simulink model "controllo_Completo_v14"  (R2025a)
settings: Solver=VariableStepAuto  StartTime=0.0  StopTime=Durata_Simulazione  MaxStep=Passo_integrazione_massimo  RelTol=1e-3
values from neighbouring files (symbols this model uses):
  C_bat_eq_rx = 1.0    (= 1)    [p_schema_completo_generale_v2.m]
  C_bat_eq_tx = 3.5    [p_schema_completo_generale_v2.m]
  C_bus_dc_dc = 1.5e-3    (= 0.0015)    [p_schema_completo_generale_v2.m]
  C_ris = 1/(w_dc_ac_nom^2*L_coil)    (= 6.49245057301e-08)    [p_schema_completo_generale_v2.m]
  dead_time_dc_dc = 0.3e-6    (= 3e-07)    [p_schema_completo_generale_v2.m]
  duty_A_0_tx = V_bat_0_tx/V_dc_0_tx    (= 0.472727272727)    [p_schema_completo_generale_v2.m]
  duty_B_0_tx = duty_A_0_tx    (= 0.472727272727)    [p_schema_completo_generale_v2.m]
  duty_leg_A_dc_dc_0_tx = V_bat_0_tx/V_dc_0_tx    (= 0.472727272727)    [p_schema_completo_generale_v2.m]
  duty_leg_B_dc_dc_0_tx = duty_leg_A_dc_dc_0_tx    (= 0.472727272727)    [p_schema_completo_generale_v2.m]
  Ibat_rif_max = 50    [p_schema_completo_generale_v2.m]
  Ibat_rif_min = -50    [p_schema_completo_generale_v2.m]
  Kp_P_tensione_batteria_rx = 1/modulo_catena_aperta_tensione_batteria_reg_P_rx    [p_schema_completo_generale_v2.m]
  Kp_P_tensione_batteria_tx = 1/modulo_catena_aperta_tensione_batteria_reg_P_tx    [p_schema_completo_generale_v2.m]
  L_coil = 54e-6    (= 5.4e-05)    [p_schema_completo_generale_v2.m]
  L_filtro_dc_dc = 65e-6    (= 6.5e-05)    [p_schema_completo_generale_v2.m]
  M_coil = k*sqrt(L_coil^2)    [p_schema_completo_generale_v2.m]
  Parametri_Controllori = [Parametri_Controllori     PI_corrente_trasm_tf_disc_den(2) PI_corrente_trasm_tf_disc_num(1) PI_corrente_trasm_tf_disc_num(2)]    [p_schema_completo_generale_v2.m]
  R_bat = 32e-3    (= 0.032)    [p_schema_completo_generale_v2.m]
  R_coil = w_dc_ac_nom*L_coil/Q_coil    (= 0.2883982056)    [p_schema_completo_generale_v2.m]
  R_coil_M = sqrt(w_dc_ac_nom^2)*M_coil/sqrt(Q_coil^2)    [p_schema_completo_generale_v2.m]
  R_Lfiltro_dc_dc = 6.5e-3    (= 0.0065)    [p_schema_completo_generale_v2.m]
  Req_Lfiltro_dc_dc = (R_Lfiltro_dc_dc+Rds_on_dc_dc)    (= 0.0075)    [p_schema_completo_generale_v2.m]
  Rshunt_coil = 1e5    (= 100000)    [p_schema_completo_generale_v2.m]
  Rshunt_Lfiltro = 1e6    (= 1000000)    [p_schema_completo_generale_v2.m]
  T_dc_ac = 1/freq_dc_ac    (= 1.17647058824e-05)    [p_schema_completo_generale_v2.m]
  T_dc_dc = 1/freq_dc_dc    (= 7.8431372549e-06)    [p_schema_completo_generale_v2.m]
  tau_filtro_anti_aliasing = R_filtro_anti_aliasing*C_filtro_anti_aliasing    (= 1.96e-06)    [p_schema_completo_generale_v2.m]
  tau_filtro_pb_coil = 1/(2*pi*f_filtro_pb_coil)    (= 3.18309886184e-05)    [p_schema_completo_generale_v2.m]
  tau_filtro_pb_corrente_bat = 1/(2*pi*f_filtro_pb_corrente_bat)    (= 2.49654812693e-05)    [p_schema_completo_generale_v2.m]
  Ts_BMS = 1e-3    (= 0.001)    [p_schema_completo_generale_v2.m]
  Ts_dc_ac = 4*T_dc_ac    (= 4.70588235294e-05)    [p_schema_completo_generale_v2.m]
  Ts_dc_dc = Ts_dc_ac    (= 4.70588235294e-05)    [p_schema_completo_generale_v2.m]
  Ts_trasmissione = 1e-3    (= 0.001)    [p_schema_completo_generale_v2.m]
  V_bat_0_rx = V_bat_nom    (= 96)    [p_schema_completo_generale_v2.m]
  V_bat_0_tx = V_bat_max-5    (= 104)    [p_schema_completo_generale_v2.m]
  V_bat_max = 109    [p_schema_completo_generale_v2.m]
  V_bat_max_alg = 218    [Controllo_tensione_bus_dc.m]    (also in Controllo_tensione_bus_dc_corrente_bobina.m; p_schema_completo_generale_v2.m)
  V_bat_min = 75    [p_schema_completo_generale_v2.m]
  V_bat_min_alg = 37.5    [Controllo_tensione_bus_dc.m]    (also in Controllo_tensione_bus_dc_corrente_bobina.m; p_schema_completo_generale_v2.m)
  V_dc_0_rx = 230    [p_schema_completo_generale_v2.m]
  V_dc_0_tx = 220    [p_schema_completo_generale_v2.m]
  Vbat_rif_max_tx = V_bat_max    (= 109)    [p_schema_completo_generale_v2.m]
  Vbat_rif_min_tx = V_bat_min    (= 75)    [p_schema_completo_generale_v2.m]
  Vdc_rif_max_tx = V_dc_nom+5    (= 255)    [p_schema_completo_generale_v2.m]
  Vdc_rif_min_tx = V_dc_nom-5    (= 245)    [p_schema_completo_generale_v2.m]
undefined symbols (not defined in the file or in its folder): Ceq_bat_tx, Cris_tx, Lfilt_dc_dc, Lfiltro_dc_dc_tx, R_bat_rx, R_bat_tx
libraries: simulink x44, spsSeriesRLCBranchLib x36, spsCurrentMeasurementLib x20, spsMosfetLib x16, spsVoltageMeasurementLib x12, simulink_extras x4, spsControlledCurrentSourceLib x4, spsControlledVoltageSourceLib x4, spsDCVoltageSourceLib x2, spsMutualInductanceLib x1, spsGroundLib x1, sps_lib x1
(part 7 of 7)

== matlab function controllo_Completo_v14/Convertitore dc-dc/Convertitore dc-dc valori medi/MATLAB Function ==
  data: Vin output; Abilitazione input; Vdc input; Vbat input; IL input; duty input
function Vin = Simula_dc_dc(Abilitazione, Vdc, Vbat, IL, duty)

    Vin=Vbat;
    
    if(Abilitazione==1)
        Vin=Vdc*duty;
    else
        if(IL>=0.01)
            Vin=Vdc;
        end
        if(IL<=-0.01)
            Vin=0;
        end
        if(abs(IL)<0.01)
            Vin=Vbat;
        end    
    end

== matlab function controllo_Completo_v14/Convertitore dc-dc/Convertitore dc-dc valori medi/MATLAB Function1 ==
  data: Vin output; Abilitazione input; Vdc input; Vbat input; IL input; duty input
function Vin = Simula_dc_dc(Abilitazione, Vdc, Vbat, IL, duty)

    Vin=Vbat;
    
    if(Abilitazione==1)
        Vin=Vdc*duty;
    else
        if(IL>=0.01)
            Vin=Vdc;
        end
        if(IL<=-0.01)
            Vin=0;
        end
        if(abs(IL)<0.01)
            Vin=Vbat;
        end    
    end
